simulink model "model_non_linear_robust"  (R2023b)
settings: Solver=VariableStepAuto  StartTime=0.0  StopTime=50  FixedStep=0.001  MaxStep=1e-2  RelTol=1e-3
undefined symbols (not defined in the file or in its folder): A, A_M, b, b_M, gamma, P, theta
settings Model: Creator=Катя  LastModifiedBy=deniskirbaba

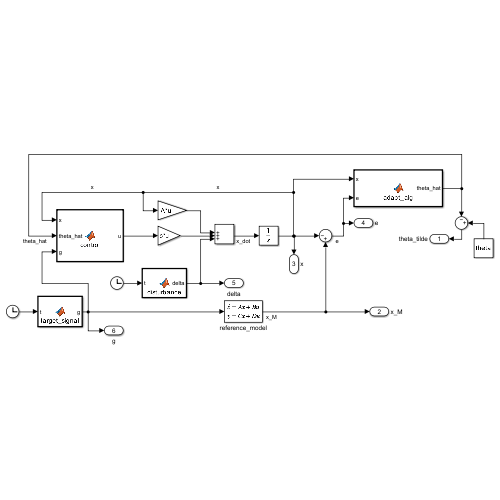
[thumbnail: Simulink's stored preview of the top-level diagram]
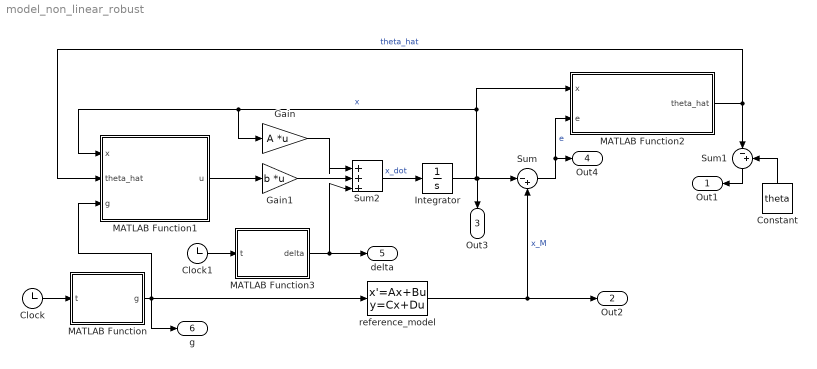
== system model_non_linear_robust ==
  Clock : Clock
  Clock1 : Clock
  Constant : Constant  Value=theta
  Gain : Gain  Gain=A  Multiplication=Matrix(K*u)
  Gain1 : Gain  Gain=b  Multiplication=Matrix(K*u)
  Integrator : Integrator
  MATLAB Function : MATLAB Function  TreatAsAtomicUnit=on
  MATLAB Function1 : MATLAB Function  TreatAsAtomicUnit=on
  MATLAB Function2 : MATLAB Function  TreatAsAtomicUnit=on
  MATLAB Function3 : MATLAB Function  TreatAsAtomicUnit=on
  Sum : Sum  Inputs=|-+
  Sum1 : Sum  Inputs=|-+
  Sum2 : Sum  Inputs=|+++
  reference_model : StateSpace  A=A_M  B=b_M  C=eye(2)  D=[0; 0]  InitialCondition=0
  Out1 : Outport  SignalName=theta_tilde
  Out2 : Outport  Port=2  SignalName=x_M
  Out3 : Outport  Port=3  SignalName=x
  Out4 : Outport  Port=4  SignalName=e
  delta : Outport  Port=5
  g : Outport  Port=6
  wires:
  reference_model/1 -> Out2/1, Sum/2  "x_M"
  Clock/1 -> MATLAB Function/1(t)
  MATLAB Function/1(g) -> g/1, MATLAB Function1/3(g), reference_model/1
  Sum/1 -> Out4/1, MATLAB Function2/2(e)  "e"
  MATLAB Function2/1(theta_hat) -> Sum1/1, MATLAB Function1/2(theta_hat)  "theta_hat"
  Constant/1 -> Sum1/2
  Gain/1 -> Sum2/1
  Gain1/1 -> Sum2/2
  Integrator/1 -> Sum/1, Out3/1, MATLAB Function2/1(x), Gain/1, MATLAB Function1/1(x)  "x"
  MATLAB Function3/1(delta) -> Sum2/3, delta/1
  Sum2/1 -> Integrator/1  "x_dot"
  MATLAB Function1/1(u) -> Gain1/1
  Clock1/1 -> MATLAB Function3/1(t)
  Sum1/1 -> Out1/1

== matlab function model_non_linear_robust/MATLAB Function1 ==
  data: x input; theta_hat input; u output; g input; kappa parameter
function u = control(x, theta_hat, g, kappa)
    u = theta_hat.' * x + g / kappa;
end

== matlab function model_non_linear_robust/MATLAB Function ==
  data: t input; g output
function g = target_signal(t)
    g = 7 * sign(cos(0.9 * t)) + 8;
end

== matlab function model_non_linear_robust/MATLAB Function2 ==
  data: x input; theta_hat output; e input; gamma parameter; b parameter; P parameter
function theta_hat = adapt_alg(x, e, gamma, b, P)
    theta_hat = gamma * x * b.' * P * e;
end

== matlab function model_non_linear_robust/MATLAB Function3 ==
  data: t input; delta output
function delta = disturbance(t)

delta = [0.6*sin(10*t)+0.1*sin(50*t);
        0.5*cos(12*t)+0.2*sin(30*t)];
